simulink model "hopsim1model"  (R2023b)
settings: Solver=VariableStepAuto  StartTime=0.0  StopTime=120  RelTol=1e-3
values from neighbouring files (symbols this model uses):
  G = [0 0 0     0 0 0    0 0 0    0 0 0]'    [hopsim1.m]    (also in hopsim2.m = [0 0   0 0   0 0 10    0 0 0]')
  g = 9.81    [hopsim1.m]    (also in hopsim2.m)
  K = round(K,5)    [hopsim1.m]    (also in hopsim2.m)
  mass = 0.627    [hopsim1.m]    (also in hopsim2.m)
  V = 5    [hopsim1.m]    (also in hopsim2.m = 1)
libraries: shared6dof x1
settings Model: Creator=jacksonwright  LastModifiedBy=jacksonwright

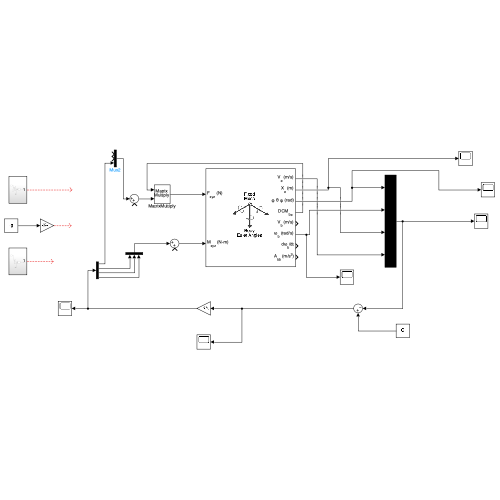
[thumbnail: Simulink's stored preview of the top-level diagram]
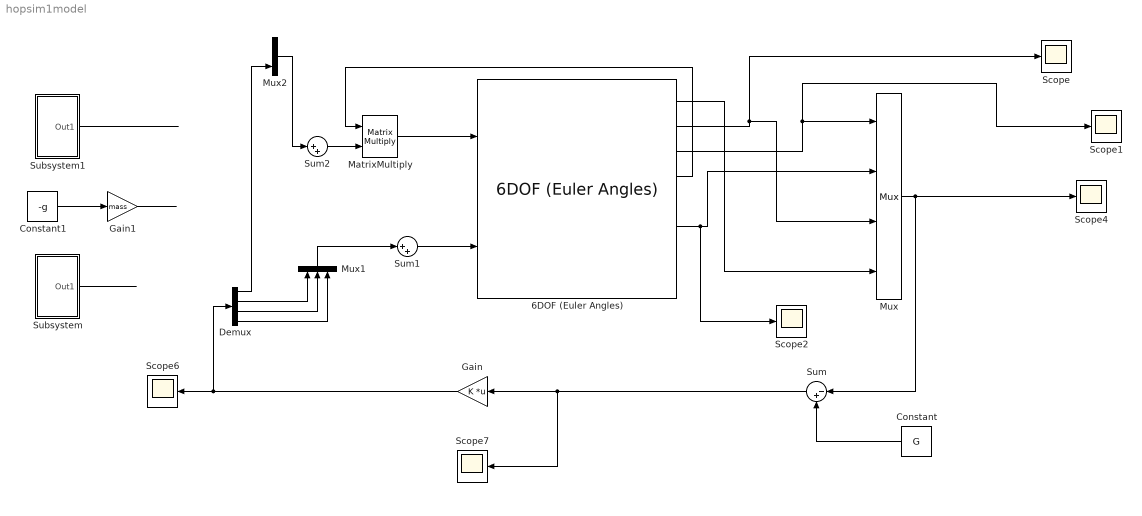
== system hopsim1model ==
  6DOF (Euler Angles) : shared6dof/6DOF (Euler Angles)  units=Metric (MKS)  mtype=Fixed  rep=Euler Angles  xme_0=[0 0 0]  Vm_0=[0 0 0]  eul_0=[0 0 0]  pm_0=[0 0 0]  mass_0=mass  mass_e=0.5  mass_f=2.0  inertia=imat  inertia_e=eye(3)  inertia_f=2*eye(3)  k_quat=1.0  vre_flag=on  abi_flag=off  aMode=0  xme_statename=''  Vm_statename=''  eul_statename=''  quat_statename=''  pm_statename=''  mass_statename=''
  Constant : Constant  Value=G
  Constant1 : Constant  Value=-g
  Demux : Demux
  Gain : Gain  Gain=K  Multiplication=Matrix(K*u)
  Gain1 : Gain  Gain=mass
  MatrixMultiply : Product  Multiplication=Matrix(*)
  Mux : Mux
  Mux1 : Mux  Inputs=3
  Mux2 : Mux  Inputs=3
  Scope{,1..2,4,6..7} (6 alike) : Scope
  Subsystem : Subsystem
  Subsystem1 : Subsystem
  Sum : Sum  Inputs=|-+
  Sum1 : Sum  Inputs=|++
  Sum2 : Sum  Inputs=|++
  wires:
  Mux/1 -> Scope4/1, Sum/1
  Constant/1 -> Sum/2
  Sum1/1 -> 6DOF (Euler Angles)/2
  6DOF (Euler Angles)/2 -> Scope/1, Mux/3
  6DOF (Euler Angles)/1 -> Mux/4
  Constant1/1 -> Gain1/1
  Gain1/1 -> ?
  6DOF (Euler Angles)/4 -> MatrixMultiply/1
  Demux/1 -> Mux2/3
  Mux2/1 -> Sum2/1
  Demux/2 -> Mux1/1
  Demux/3 -> Mux1/2
  6DOF (Euler Angles)/6 -> Scope2/1, Mux/2
  6DOF (Euler Angles)/3 -> Scope1/1, Mux/1
  Mux1/1 -> Sum1/1
  Subsystem1/1(Out1) -> ?
  MatrixMultiply/1 -> 6DOF (Euler Angles)/1
  Sum2/1 -> MatrixMultiply/2
  Sum/1 -> Scope7/1, Gain/1
  Gain/1 -> Demux/1, Scope6/1
  Subsystem/1(Out1) -> ?
  Demux/4 -> Mux1/3

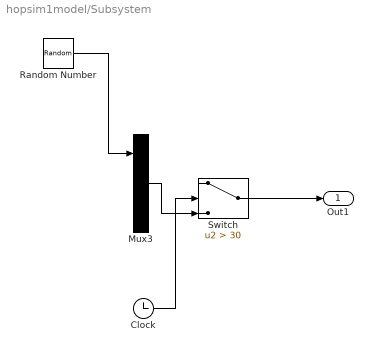
== system hopsim1model/Subsystem ==
  Clock : Clock
  Mux3 : Mux  Inputs=3
  Random Number : RandomNumber  Variance=V  SampleTime=3
  Switch : Switch  Criteria=u2 > Threshold  Threshold=30  SaturateOnIntegerOverflow=off  InputSameDT=off
  Out1 : Outport
  wires:
  Switch/1 -> Out1/1
  Random Number/1 -> Mux3/1
  Clock/1 -> Switch/2
  Mux3/1 -> Switch/3

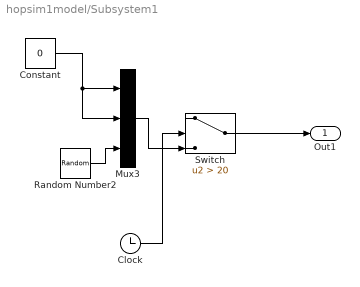
== system hopsim1model/Subsystem1 ==
  Clock : Clock
  Constant : Constant  Value=0
  Mux3 : Mux  Inputs=3
  Random Number2 : RandomNumber  Variance=V  SampleTime=3
  Switch : Switch  Criteria=u2 > Threshold  Threshold=20  SaturateOnIntegerOverflow=off  InputSameDT=off
  Out1 : Outport
  wires:
  Switch/1 -> Out1/1
  Constant/1 -> Mux3/1, Mux3/2
  Random Number2/1 -> Mux3/3
  Clock/1 -> Switch/2
  Mux3/1 -> Switch/3
